simulink model "LEDBlinkTwoLEDs_model"  (R2024a)
settings: Solver=FixedStepAuto  StartTime=0.0  StopTime=tFinal  FixedStep=T  RelTol=1e-3  EnableMultiTasking=on
values from neighbouring files (symbols this model uses):
  repeatingPulsePeriod = 1    [MAIN_LEDBlinkTwoLEDs.m]    (also in Step01_LEDBlinkTwoLEDs.m)
  repeatingPulseWidthPercent = 50    [MAIN_LEDBlinkTwoLEDs.m]    (also in Step01_LEDBlinkTwoLEDs.m = 70)
libraries: arduinolib x2
settings Model: SimulationMode=external  ExtModeTrigDuration=2  Creator=Christopher  LastModifiedBy=chris
settings SolverCC: AlgebraicLoopSolver=TrustRegion  AutoInsertRateTranBlk=on
settings DataIOCC: LimitDataPoints=on  StreamToWorkspace=on  ReturnWorkspaceOutputs=off
settings OptimizationCC: LifeSpan=1  MaxStackSize=64
settings DebuggingCC: UnconnectedInputMsg=warning  UnconnectedOutputMsg=warning  UnconnectedLineMsg=warning  AllowSymbolicDim=off  SFUnexpectedBacktrackingDiag=warning  SFNoUnconditionalDefaultTransitionDiag=warning  SFExecutionAtInitializationDiag=none  ArithmeticOperatorsInVariantConditions=warning
settings HardwareCC: ProdBitPerInt=16  ProdBitPerPointer=16  ProdBitPerSizeT=16  ProdBitPerPtrDiffT=16  ProdLargestAtomicFloat=None  ProdWordSize=8  ProdHWDeviceType=Atmel->AVR
settings ModelReferenceCC: EnableRefExpFcnMdlSchedulingChecks=on  PropagateSignalLabelsOutOfModel=off
settings SFSimCC: SimUseLocalCustomCode=off  CustomCodeUndefinedFunction=UseInterfaceOnly
settings RTWCC: Description=Embedded Coder  SystemTargetFile=ert.tlc  HardwareBoard=Arduino Nano 3.0  TemplateMakefile=ert_default_tmf  RTWVerbose=off  RTWUseLocalCustomCode=off  Toolchain=Arduino AVR  BuildConfiguration=Faster Runs  GPUComputeCapability=3.5
settings CodeAppCC: MangleLength=10  StateflowObjectComments=on
settings ERTTargetCC: MultiwordLength=2048  ERTCustomFileBanners=off  SupportContinuousTime=on  SupportNonInlinedSFcns=on  RemoveResetFunc=off  SupportVariableSizeSignals=on  ModelStepFunctionPrototypeControlCompliant=off  ExtMode=on  ExtModeTransport=3  ExtModeStaticAlloc=on  ExtModeAutomaticAllocSize=off  ExtModeStaticAllocSize=250  ExtModeMexFile=ext_xcp  ExtModeMexArgs='127.0.0.1' 0 17725  ExtModeIntrfLevel=Level2 - Open  ERTSrcFileBannerTemplate=codertarget_code_template.cgt  ERTHdrFileBannerTemplate=codertarget_code_template.cgt  ERTDataSrcFileTemplate=codertarget_code_template.cgt  ERTDataHdrFileTemplate=codertarget_code_template.cgt  ConvertIfToSwitch=off  SuppressUnreachableDefaultCases=off
settings ConfigComp: CovMetricSettings=dw  CovSaveCumulativeToWorkspaceVar=on  CovSaveSingleToWorkspaceVar=on  CovExternalEMLEnable=off

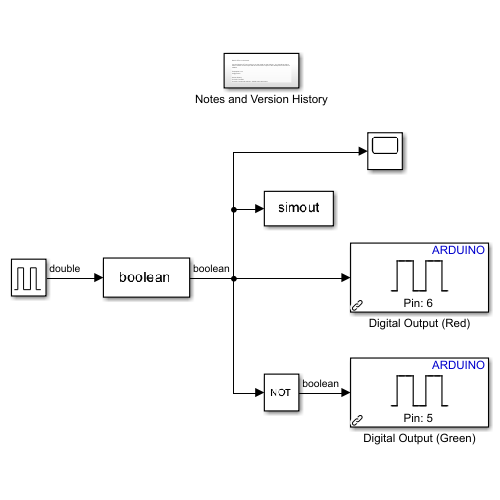
[thumbnail: Simulink's stored preview of the top-level diagram]
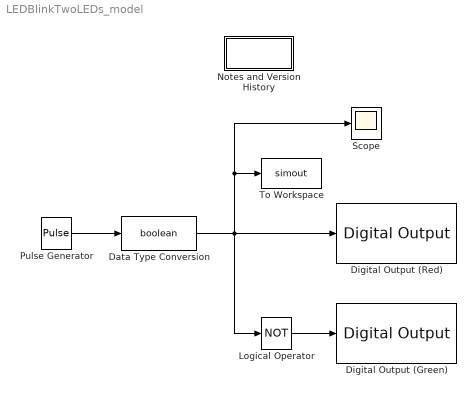
== system LEDBlinkTwoLEDs_model ==
  Data Type Conversion : DataTypeConversion  OutDataTypeStr=boolean  SaturateOnIntegerOverflow=off  RndMeth=Floor
  Digital Output (Green) : arduinolib/Digital Output  pinNumber=PinLED_G  Direction=output  blockPlatform=arduino
  Digital Output (Red) : arduinolib/Digital Output  pinNumber=PinLED_R  Direction=output  blockPlatform=arduino
  Logical Operator : Logic  Operator=NOT  AllPortsSameDT=off  OutDataTypeStr=boolean
  Notes and Version History : Subsystem
  Pulse Generator : DiscretePulseGenerator  PulseType=Time based  Period=repeatingPulsePeriod  PulseWidth=repeatingPulseWidthPercent
  Scope : Scope
  To Workspace : ToWorkspace  VariableName=simout  SaveFormat=Structure With Time  SampleTime=-1
  wires:
  Data Type Conversion/1 -> Digital Output (Red)/1, Scope/1, To Workspace/1, Logical Operator/1
  Pulse Generator/1 -> Data Type Conversion/1
  Logical Operator/1 -> Digital Output (Green)/1

== system LEDBlinkTwoLEDs_model/Notes and Version History ==
  note: Blink 2 LEDs on the board.
      |
      | Use the 'Monitor & Tune' option to run the model on the Arduino. You should be able to see the results on the scope and the result will be output to the Workspace in the simout variable.
      |
      | Christopher Lum
      | lum@uw.edu
      |
      | Version History
      | 12/13/24: Created
      | 12/14/24: Continued working. Added scope and notes.
